simulink model "triad_simple_test"  (R2016b)
settings: Solver=VariableStepAuto  StartTime=0.0  StopTime=50  RelTol=1e-3
values from neighbouring files (symbols this model uses):
  fsw_params = init_fsw_params()    [init_ctrl_TRIAD_test.m]
  mag_vec_init = mag_vec_init/norm(mag_vec_init)    [ctrl_TRIAD_test.m]    (also in init_ctrl_TRIAD_test.m; init_triad_simple_test.m; triad_simple_test_script.m)
  quat_init = quat_init./norm(quat_init)    [init_triad_simple_test.m]    (also in triad_simple_test_script.m = [cos(0.5*thet) sin(0.5*thet)/sqrt(3)* ones(1,3)]')
  sun_vec_init = sun_vec_init/norm(sun_vec_init)    [ctrl_TRIAD_test.m]    (also in init_ctrl_TRIAD_test.m; init_triad_simple_test.m; triad_simple_test_script.m)
libraries: dspmathops x6, vrlib x4
settings Model: Creator=sexymathemagician  LastModifiedBy=sexymathemagician

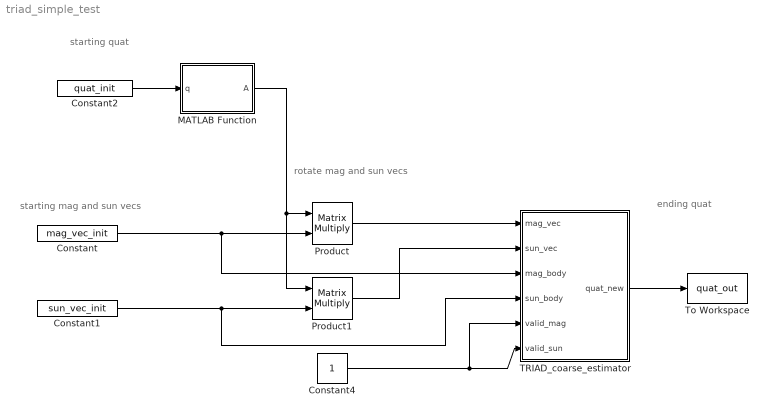
== system triad_simple_test ==
  note: rotate mag and sun vecs
  note: starting mag and sun vecs
  note: ending quat
  note: starting quat
  Constant : Constant  Value=mag_vec_init
  Constant1 : Constant  Value=sun_vec_init
  Constant2 : Constant  Value=quat_init
  Constant4 : Constant
  MATLAB Function : MATLAB Function  TreatAsAtomicUnit=on
  Product : Product  Multiplication=Matrix(*)
  Product1 : Product  Multiplication=Matrix(*)
  TRIAD_coarse_estimator : Subsystem
  To Workspace : ToWorkspace  VariableName=quat_out  SaveFormat=Timeseries  SampleTime=-1
  wires:
  Constant2/1 -> MATLAB Function/1(q)
  MATLAB Function/1(A) -> Product1/1, Product/1
  Constant/1 -> TRIAD_coarse_estimator/3(mag_body), Product/2
  Constant1/1 -> TRIAD_coarse_estimator/4(sun_body), Product1/2
  Constant4/1 -> TRIAD_coarse_estimator/6(valid_sun), TRIAD_coarse_estimator/5(valid_mag)
  TRIAD_coarse_estimator/1(quat_new) -> To Workspace/1
  Product/1 -> TRIAD_coarse_estimator/1("mag_vec ")
  Product1/1 -> TRIAD_coarse_estimator/2("sun_vec ")

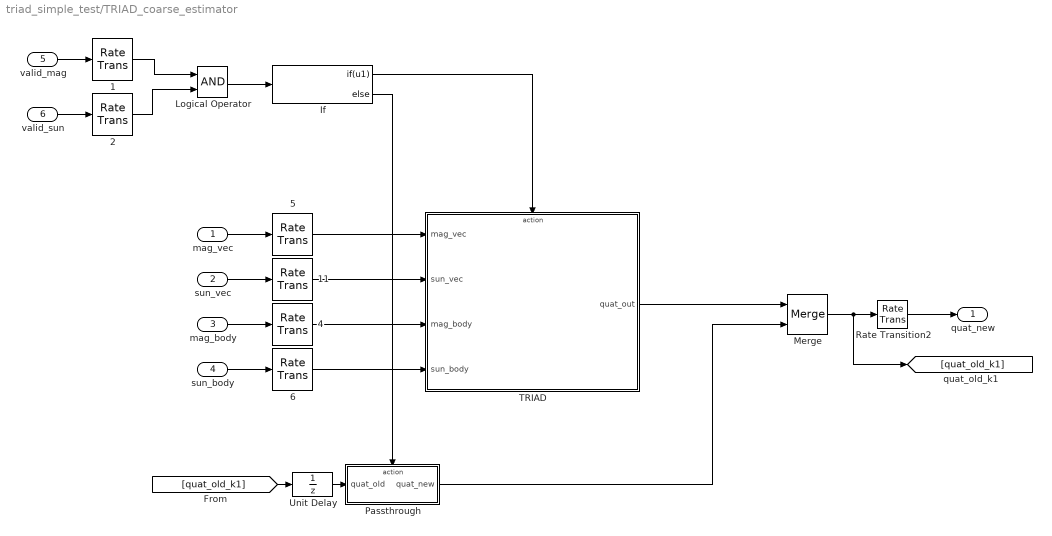
== system triad_simple_test/TRIAD_coarse_estimator ==
  "mag_vec " : Inport
  "sun_vec " : Inport  Port=2
  mag_body : Inport  Port=3
  sun_body : Inport  Port=4
  valid_mag : Inport  Port=5
  valid_sun : Inport  Port=6
  " 1" : RateTransition  X0=fsw_params.estimation.ic.rt_valid_mag  OutPortSampleTime=fsw_params.estimation.sample_time_s
  " 11" : RateTransition  X0=fsw_params.estimation.ic.rt_sun_eci_est  OutPortSampleTime=fsw_params.estimation.sample_time_s
  " 2" : RateTransition  X0=fsw_params.estimation.ic.rt_valid_sun  OutPortSampleTime=fsw_params.estimation.sample_time_s
  " 4" : RateTransition  X0=fsw_params.estimation.ic.rt_mag_body  OutPortSampleTime=fsw_params.estimation.sample_time_s
  " 5" : RateTransition  X0=fsw_params.estimation.ic.rt_mag_eci_est  OutPortSampleTime=fsw_params.estimation.sample_time_s
  " 6" : RateTransition  X0=fsw_params.estimation.ic.rt_sun_body  OutPortSampleTime=fsw_params.estimation.sample_time_s
  If : If  IfExpression=u1
  Logical Operator : Logic  AllPortsSameDT=off  OutDataTypeStr=boolean
  Merge : Merge
  Passthrough : Subsystem  TreatAsAtomicUnit=on
  Rate Transition2 : RateTransition  X0=fsw_params.estimation.ic.quat_est_init
  "TRIAD " : Subsystem  TreatAsAtomicUnit=on
  Unit Delay : UnitDelay  InitialCondition=fsw_params.estimation.ic.quat_est_init  SampleTime=fsw_params.estimation.sample_time_s
  quat_new : Outport
  wires:
  "mag_vec "/1 -> " 5"/1
  "sun_vec "/1 -> " 11"/1
  mag_body/1 -> " 4"/1
  sun_body/1 -> " 6"/1
  If/1 -> "TRIAD "/Action
  If/2 -> Passthrough/Action
  "TRIAD "/1("quat_out ") -> Merge/1
  Passthrough/1(quat_new) -> Merge/2
  Merge/1 -> [quat_old_k1], Rate Transition2/1
  valid_mag/1 -> " 1"/1
  valid_sun/1 -> " 2"/1
  Logical Operator/1 -> If/1
  Rate Transition2/1 -> quat_new/1
  " 1"/1 -> Logical Operator/1
  " 2"/1 -> Logical Operator/2
  " 4"/1 -> "TRIAD "/3(mag_body)
  " 6"/1 -> "TRIAD "/4(sun_body)
  " 11"/1 -> "TRIAD "/2("sun_vec ")
  " 5"/1 -> "TRIAD "/1("mag_vec ")
  [quat_old_k1] -> Unit Delay/1
  Unit Delay/1 -> Passthrough/1(quat_old)

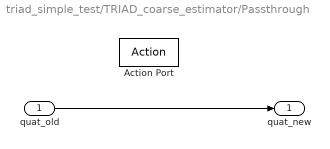
== system triad_simple_test/TRIAD_coarse_estimator/Passthrough ==
  quat_old : Inport
  Action Port : ActionPort  ActionType=else
  quat_new : Outport
  wires:
  quat_old/1 -> quat_new/1

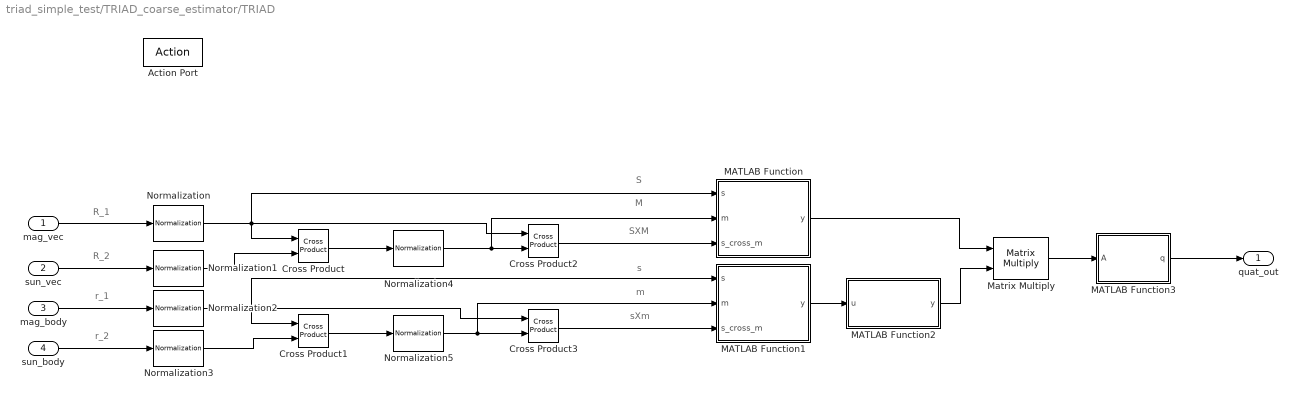
== system triad_simple_test/TRIAD_coarse_estimator/TRIAD  ==
  note: sXm
  note: SXM
  note: s
  note: S
  note: m
  note: M
  note: R_2
  note: R_1
  note: r_2
  note: r_1
  "mag_vec " : Inport
  "sun_vec " : Inport  Port=2
  mag_body : Inport  Port=3
  sun_body : Inport  Port=4
  Action Port : ActionPort  ActionType=then
  Cross Product{,1..3} (4 alike) : vrlib/Utilities/Cross Product
  MATLAB Function : MATLAB Function  TreatAsAtomicUnit=on
  MATLAB Function1 : MATLAB Function  TreatAsAtomicUnit=on
  MATLAB Function2 : MATLAB Function  TreatAsAtomicUnit=on
  MATLAB Function3 : MATLAB Function  TreatAsAtomicUnit=on
  Matrix Multiply : Product  Multiplication=Matrix(*)
  Normalization{,1..5} (6 alike) : dspmathops/Normalization  NormType=2-norm  Bias=1e-10  NormOver=Each column  Dimension=1  outputDataTypeStr=Inherit: Same as product output  outputLastDataTypeStr=Inherit: Same as product output  outputMin=[]  outputMax=[]  accumDataTypeStr=Inherit: Same as product output  accumLastDataTypeStr=Inherit: Same as product output  roundingMode=Floor  overflowMode=off
  "quat_out " : Outport
  wires:
  "mag_vec "/1 -> Normalization/1
  "sun_vec "/1 -> Normalization1/1
  mag_body/1 -> Normalization2/1
  sun_body/1 -> Normalization3/1
  Normalization1/1 -> Cross Product/2
  Normalization2/1 -> Cross Product3/1, MATLAB Function1/1(s), Cross Product1/1
  Normalization3/1 -> Cross Product1/2
  Cross Product/1 -> Normalization4/1
  Cross Product1/1 -> Normalization5/1
  Normalization4/1 -> MATLAB Function/2(m), Cross Product2/2
  Normalization5/1 -> MATLAB Function1/2(m), Cross Product3/2
  Cross Product2/1 -> MATLAB Function/3(s_cross_m)
  Cross Product3/1 -> MATLAB Function1/3(s_cross_m)
  MATLAB Function1/1(y) -> MATLAB Function2/1(u)
  MATLAB Function/1(y) -> Matrix Multiply/1
  MATLAB Function2/1(y) -> Matrix Multiply/2
  MATLAB Function3/1(q) -> "quat_out "/1
  Matrix Multiply/1 -> MATLAB Function3/1(A)
  Normalization/1 -> Cross Product/1, Cross Product2/1, MATLAB Function/1(s)

== matlab function triad_simple_test/MATLAB Function ==
  data: q input; A output
function A = quatToMatrix(q)
%#codegen

eta = q(1);
eps = q(2:4);

A = (2*eta^2 -1)*eye(3) + 2*(eps*eps') - 2*eta*skew(eps);


end

function cross = skew(a)
%#codegen

cross = [0 -a(3) a(2);
         a(3) 0 -a(1);
        -a(2) a(1) 0];

end

== matlab function triad_simple_test/TRIAD_coarse_estimator/TRIAD /MATLAB Function ==
  data: s input; y output; m input; s_cross_m input
function y = vecStackCols(s, m, s_cross_m)
%#codegen

% stacks the 3x1 vectors s, m and s_cross_m into a 3x3 matrix y = [s|m|sXm]

y = [s m s_cross_m];
end

== matlab function triad_simple_test/TRIAD_coarse_estimator/TRIAD /MATLAB Function1 ==
  data: s input; y output; m input; s_cross_m input
function y = vecStackCols(s, m, s_cross_m)
%#codegen

% stacks the 3x1 vectors s, m and s_cross_m into a 3x3 matrix y = [s|m|sXm]

y = [s m s_cross_m];
end

== matlab function triad_simple_test/TRIAD_coarse_estimator/TRIAD /MATLAB Function2 ==
  data: u input; y output
function y = matrixTranspose(u)
%#codegen

y = u';

== matlab function triad_simple_test/TRIAD_coarse_estimator/TRIAD /MATLAB Function3 ==
  data: A input; q output
function q = attitudeToQuat(A)
%#codegen
% converts the proper orthogonal matrix A into a (scalar-first) quaternion

qw = 0.5*sqrt(1 + A(1,1) + A(2,2) + A(3,3));
qx = (A(3,2) - A(2,3))/( 4 *qw);
qy = (A(1,3) - A(3,1))/( 4 *qw);
qz = (A(2,1) - A(1,2))/( 4 *qw);

q = [qw qx qy qz]';



end
